simulink model "PodizacNapona"  (R2014b)
settings: Solver=ode23tb  StartTime=0.0  StopTime=0.2  MaxStep=Tsim  RelTol=1e-4
values from neighbouring files (symbols this model uses):
  C = 1000e-6    (= 0.001)    [MFajl.m]
  L = 120e-6    (= 0.00012)    [MFajl.m]
  R = 10    [MFajl.m]
  Ts = 1/fs    (= 5e-05)    [MFajl.m]
  Vg = 12    [MFajl.m]
libraries: powerlib x15, simulink x1
settings Model: Creator=Zorana  LastModifiedBy=Zorana

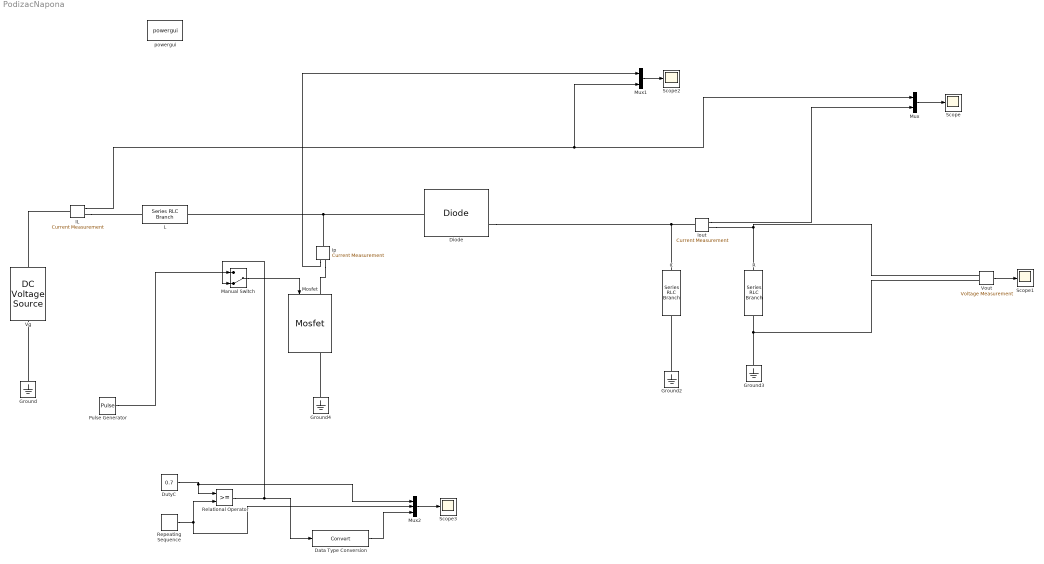
== system PodizacNapona ==
  C : powerlib/Elements/Series RLC Branch  LConnTagsString=__new0  RConnTagsString=__new0  BranchType=C  Resistance=1  Inductance=L  SetiL0=off  InitialCurrent=0  Capacitance=C  Setx0=off  InitialVoltage=0  Measurements=None
  Data Type Conversion : DataTypeConversion
  Diode : powerlib/Power Electronics/Diode  Ron=1e-6  Lon=0  Vf=0  IC=0  UseSnubber=off  Rs=500  Cs=250e-9  Measurements=on
  DutyC : Constant  Value=0.7
  Ground{,2..4} (4 alike) : powerlib/Elements/Ground  LConnTagsString=a
  IL : powerlib/Measurements/Current Measurement  PhasorSimulation=off  OutputType=Complex  PSBequivalent=0
  Iout : powerlib/Measurements/Current Measurement  PhasorSimulation=off  OutputType=Complex  PSBequivalent=0
  Ip : powerlib/Measurements/Current Measurement  PhasorSimulation=off  OutputType=Complex  PSBequivalent=0
  L : powerlib/Elements/Series RLC Branch  LConnTagsString=__new0  RConnTagsString=__new0  BranchType=L  Resistance=1  Inductance=L  SetiL0=off  InitialCurrent=0  Capacitance=1e-6  Setx0=off  InitialVoltage=0  Measurements=None
  Manual Switch : ManualSwitch  CurrentSetting=0
  Mosfet : powerlib/Power Electronics/Mosfet  Ron=1e-6  Lon=0  Rd=1e-6  Vfd=0  IC=0  Rs=1e5  Cs=inf  Measurements=on
  Mux : Mux  Inputs=2
  Mux1 : Mux  Inputs=2
  Mux2 : Mux  Inputs=3
  Pulse Generator : DiscretePulseGenerator  PulseType=Time based  Period=Ts  PulseWidth=40
  R : powerlib/Elements/Series RLC Branch  LConnTagsString=__new0  RConnTagsString=__new0  BranchType=R  Resistance=R  Inductance=L  SetiL0=off  InitialCurrent=0  Capacitance=1e-6  Setx0=off  InitialVoltage=0  Measurements=None
  Relational Operator : RelationalOperator  OutDataTypeStr=boolean
  Repeating Sequence : simulink/Sources/Repeating Sequence  rep_seq_t=[0 Ts]  rep_seq_y=[0 1]
  Scope{,1..3} (4 alike) : Scope
      Scope2 settings: SaveName=ScopeData2
      Scope3 settings: SaveName=ScopeData3
  Vg : powerlib/Electrical Sources/DC Voltage Source  Amplitude=Vg  Measurements=None
  Vout : powerlib/Measurements/Voltage Measurement  PhasorSimulation=off  OutputType=Complex  PSBequivalent=0
  powergui : powerlib/powergui  Priority=1  SimulationMode=Continuous  SolverType=Tustin/Backward Euler (TBE)  SampleTime=50e-6  frequency=60  SPID=off  DisableSnubberDevices=off  DisableRonSwitches=off  DisableVfSwitches=off  SwTol=0  DisplayEquations=off  Interpol=off  methode=off  Ts=100  frequencyindice=0  Pbase=100e6  ErrMax=1e-4  Iterations=50  UnitsV=kV  UnitsW=MW  FunctionMessages=off  echomessages=off  HookPort=off  EnableUseOfTLC=off  x0status=blocks  RestoreLinks=warning  ResistiveCurrentMeasurement=off  Frange=[0:2:500]  Ylog=off  Xlog=on  ShowGrid=off  save=off  variable=ZData  structure=0  ZoomFFT=off  StartTime=0.0  cycles=1  DisplayStyle=1  fundamental=60  FreqAxis=off  MaxFrequency=1000  frequencyindicesteady=1  RmsSteady=1  display=off
  wires:
  Mux/1 -> Scope/1
  Vout/1 -> Scope1/1
  Mux1/1 -> Scope2/1
  Relational Operator/1 -> Manual Switch/2, Data Type Conversion/1
  DutyC/1 -> Mux2/1, Relational Operator/1
  Repeating Sequence/1 -> Relational Operator/2, Mux2/2
  Mux2/1 -> Scope3/1
  Data Type Conversion/1 -> Mux2/3
  Iout/1 -> Mux/2
  IL/1 -> Mux1/2, Mux/1
  Ip/1 -> Mux1/1
  Manual Switch/1 -> Mosfet/1
  Pulse Generator/1 -> Manual Switch/1
  connections:
  Ground/LConn1 -- Vg/LConn1
  Ground2/LConn1 -- C/RConn1
  Ground3/LConn1 -- Vout/LConn2 -- R/RConn1
  Diode/LConn1 -- Ip/LConn1 -- L/RConn1
  Diode/RConn1 -- Iout/LConn1 -- C/LConn1
  Ground4/LConn1 -- Mosfet/RConn1
  R/LConn1 -- Iout/RConn1 -- Vout/LConn1
  Vg/RConn1 -- IL/LConn1
  IL/RConn1 -- L/LConn1
  Ip/RConn1 -- Mosfet/LConn1
